simulink model "TVLQR2_sim"  (R2024b)
settings: Solver=FixedStepDiscrete  StartTime=0.0  StopTime=11380*50  FixedStep=1  RelTol=1e-3
values from neighbouring files (symbols this model uses):
  Ad = sys_d.A    [TVLQR2.m]    (also in TVLQR_dist.m)
  Bd = sys_d.B    [TVLQR2.m]    (also in TVLQR_dist.m)
  Cd = sys_d.C    [TVLQR2.m]    (also in TVLQR_dist.m)
  Dd = sys_d.D    [TVLQR2.m]    (also in TVLQR_dist.m)
  dt_sim = 0.1    [TVLQR2.m]    (also in TVLQR_dist.m)
  K_tv = zeros(3,6,N_orbit)    [TVLQR2.m]    (also in TVLQR_dist.m)
  m_max_pss = 0.166    [TVLQR2.m]    (also in TVLQR_dist.m)
  N_orbit = round(T_total / dt_sim)    [TVLQR2.m]    (also in TVLQR_dist.m)
  T_total = length(t_trim)*dt_data    [Bdot_run.m]    (also in TVLQR2.m = length(t_tv_trimmed) * dt_data; TVLQR_dist.m = length(t_tv_trimmed) * dt_data)
settings Model: Creator=zalak  LastModifiedBy=zalak

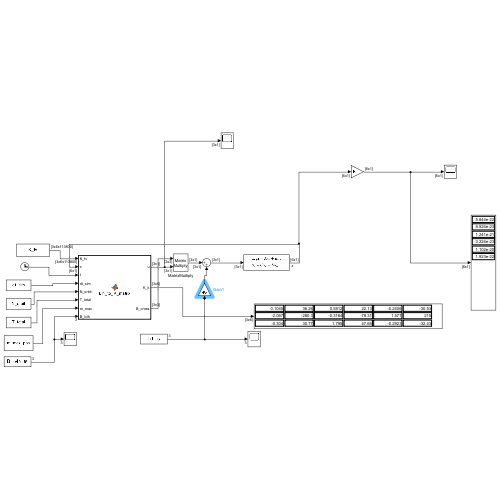
[thumbnail: Simulink's stored preview of the top-level diagram]
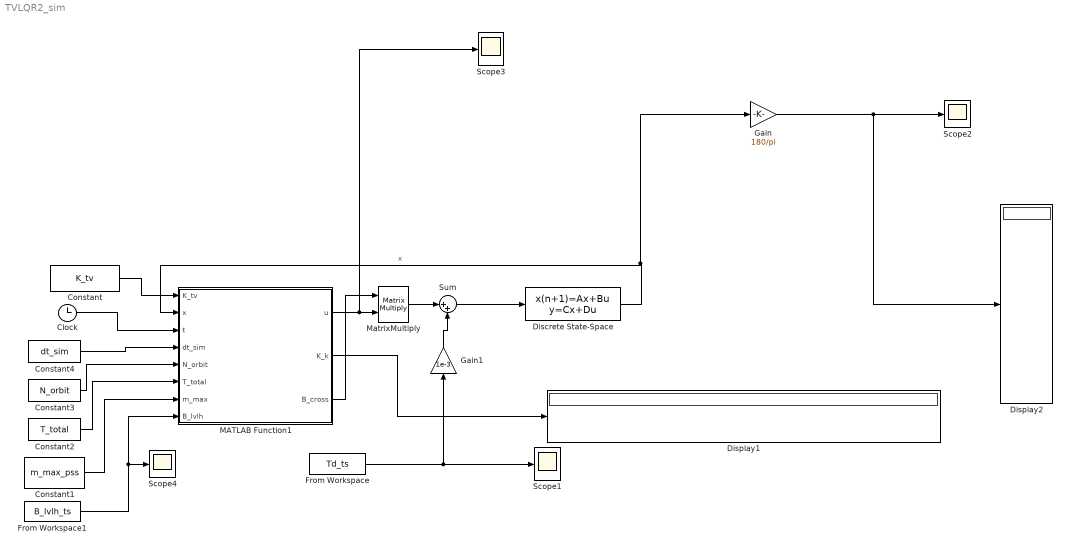
== system TVLQR2_sim ==
  Clock : Clock
  Constant : Constant  Value=K_tv
  Constant1 : Constant  Value=m_max_pss
  Constant2 : Constant  Value=T_total
  Constant3 : Constant  Value=N_orbit
  Constant4 : Constant  Value=dt_sim
  Discrete State-Space : DiscreteStateSpace  A=Ad  B=Bd  C=Cd  D=Dd  InitialCondition=[1*pi/180;0;0;0;0;0]
  Display1 : Display
  Display2 : Display
  From Workspace : FromWorkspace  VariableName=Td_ts
  From Workspace1 : FromWorkspace  VariableName=B_lvlh_ts  SampleTime=1
  Gain : Gain  Gain=180/pi
  Gain1 : Gain  Gain=1e-3
  MATLAB Function1 : MATLAB Function  TreatAsAtomicUnit=on
  MatrixMultiply : Product  Multiplication=Matrix(*)
  Scope{1..4} (4 alike) : Scope
  Sum : Sum  Inputs=|++
  wires:
  Gain/1 -> Display2/1, Scope2/1
  From Workspace1/1 -> MATLAB Function1/8(B_lvlh), Scope4/1
  MATLAB Function1/2(K_k) -> Display1/1
  MATLAB Function1/1(u) -> Scope3/1, MatrixMultiply/2
  MATLAB Function1/3(B_cross) -> MatrixMultiply/1
  MatrixMultiply/1 -> Sum/1
  From Workspace/1 -> Scope1/1, Gain1/1
  Sum/1 -> Discrete State-Space/1
  Constant/1 -> MATLAB Function1/1(K_tv)
  Discrete State-Space/1 -> MATLAB Function1/2(x), Gain/1  "x"
  Clock/1 -> MATLAB Function1/3(t)
  Constant1/1 -> MATLAB Function1/7(m_max)
  Constant2/1 -> MATLAB Function1/6(T_total)
  Constant3/1 -> MATLAB Function1/5(N_orbit)
  Constant4/1 -> MATLAB Function1/4(dt_sim)
  Gain1/1 -> Sum/2

== matlab function TVLQR2_sim/MATLAB Function1 ==
  data: K_tv input; x input; t input; dt_sim input; N_orbit input; T_total input; m_max input; B_lvlh input; u output; K_k output; B_cross output
function [u, K_k, B_cross] = lvlh_to_K_matrix(K_tv, x, t, dt_sim, N_orbit, T_total, m_max, B_lvlh)

% K_tv:    3×6×N_orbit lookup table (passed from workspace as constant)
% x:       6×1 state
% t:       current simulation time (from Clock block)
% dt_sim:  design grid (0.1s)
% N_orbit: number of design steps per orbit
% T_total: orbital period in seconds

phi = x(1); theta = x(3); psi = x(5);

Rx = [1,0,0; 0,cos(phi),sin(phi); 0,-sin(phi),cos(phi)];
Ry = [cos(theta),0,-sin(theta); 0,1,0; sin(theta),0,cos(theta)];
Rz = [cos(psi),sin(psi),0; -sin(psi),cos(psi),0; 0,0,1];
B_body = Rz*Ry*Rx * B_lvlh(:);

bx = B_body(1); by = B_body(2); bz = B_body(3);
B_cross = [0,bz,-by; -bz,0,bx; by,-bx,0];

% Find current index in the periodic schedule
t_mod = mod(t, T_total);
k = floor(t_mod / dt_sim) + 1;
k = min(max(k, 1), N_orbit);

K_k = K_tv(:,:,k);
u_nom = -0.9757 * K_k * x;

% Saturate (Psiaki proportional)
beta = max(abs(u_nom) / m_max);
if beta <= 1
    u = u_nom;
else
    u = u_nom / beta;
end
end
